simulink model "typMPC"  (R2019b)
settings: Solver=VariableStepAuto  StartTime=0.0  StopTime=10.0  RelTol=1e-3
settings Model: Creator=Daniel  LastModifiedBy=Daniel

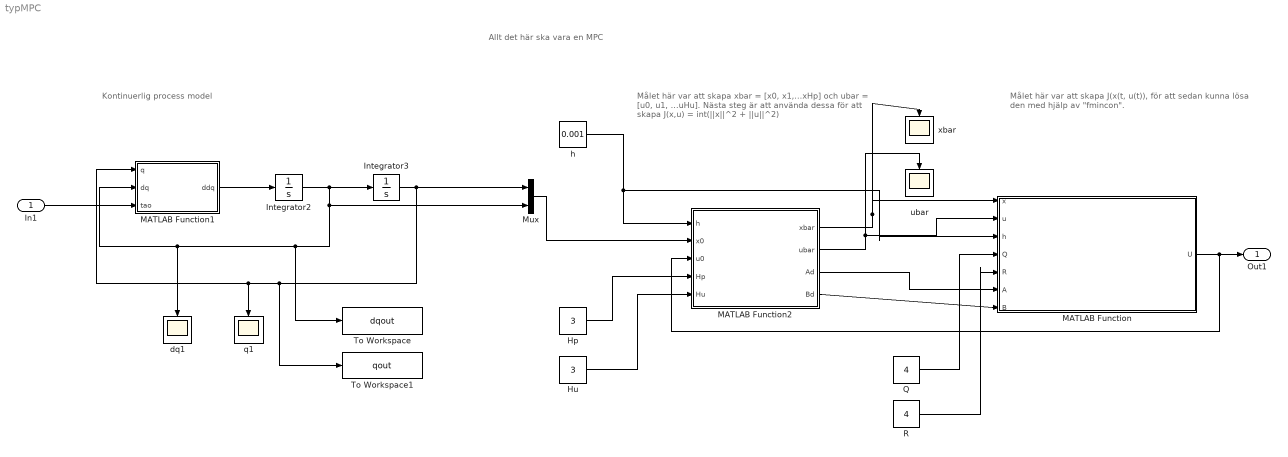
== system typMPC ==
  note: Allt det här ska vara en MPC
  note: Målet här var att skapa J(x(t, u(t)), för att sedan
      | kunna lösa den med hjälp av "fmincon".
  note: Målet här var att skapa xbar = [x0, x1,...xHp]
      | och ubar = [u0, u1, ...uHu].
      | Nästa steg är att använda dessa för att skapa
      | J(x,u) = int(||x||^2 + ||u||^2)
  note: Kontinuerlig process model
  In1 : Inport
  "Hp " : Constant  Value=3
  "Hu " : Constant  Value=3
  Integrator2 : Integrator  InitialCondition=[0;pi/6]
  Integrator3 : Integrator  InitialCondition=[0;0]
  MATLAB Function : MATLAB Function  TreatAsAtomicUnit=on
  MATLAB Function1 : MATLAB Function  TreatAsAtomicUnit=on
  MATLAB Function2 : MATLAB Function  TreatAsAtomicUnit=on
  Mux : Mux  Inputs=2
  Q : Constant  Value=4
  R : Constant  Value=4
  To Workspace : ToWorkspace  VariableName=dqout  SaveFormat=Timeseries  SampleTime=-1
  To Workspace1 : ToWorkspace  VariableName=qout  SampleTime=-1
  dq1 : Scope
  h : Constant  Value=0.001
  q1 : Scope
  ubar : Scope
  xbar : Scope
  Out1 : Outport
  wires:
  MATLAB Function2/2(ubar) -> MATLAB Function/2(u), ubar/1
  Mux/1 -> MATLAB Function2/2(x0)
  "Hu "/1 -> MATLAB Function2/5(Hu)
  MATLAB Function2/1(xbar) -> MATLAB Function/1(x), xbar/1
  "Hp "/1 -> MATLAB Function2/4(Hp)
  h/1 -> MATLAB Function/3(h), MATLAB Function2/1(h)
  Integrator3/1 -> Mux/1, To Workspace1/1, MATLAB Function1/1(q), q1/1
  MATLAB Function1/1(ddq) -> Integrator2/1
  Integrator2/1 -> Mux/2, To Workspace/1, MATLAB Function1/2(dq), dq1/1, Integrator3/1
  MATLAB Function2/3(Ad) -> MATLAB Function/6(A)
  MATLAB Function2/4(Bd) -> MATLAB Function/7(B)
  Q/1 -> MATLAB Function/4(Q)
  R/1 -> MATLAB Function/5(R)
  MATLAB Function/1(U) -> MATLAB Function2/3(u0), Out1/1
  In1/1 -> MATLAB Function1/3(tao)

== matlab function typMPC/MATLAB Function1 ==
  data: q input; ddq output; dq input; tao input
function  ddq  = testing(q,dq,tao)
%% q= [phi, theta],   dq = [dphi, dtheta]
% tao2=[0;tao];
phi = q(1,1);
theta = q(2,1);
dphi = dq(1,1);
dtheta = dq(2,1);
%Given parameters - "competition.pdf"
la  = 75*10^-3;       %[m]      - Length of arm
r  = 43*10^-3;       %[m]      - Base radius
lp  = 31.5*10^-3;     %[m]      - Length of pendulum
J  = 125*10^-6;      %[kgm^2]  - Base moment of inertia
g  = 9.8;            %[m/s^2]  - Gravity
Jc = 2.55*10^-6;     %[kgm^2]  - Moment of inertia of pendulum around c.o.m
M  = 5.44*10^-3;     %[kg]     - Mass of pendulum point mass
Jp = 7.95*10^-6;     %[kgm^2]  - Moment of inertia of pend around pivot

%Still unknown - Try to guess these as a first step
ma = 10*10^-3;       %[kg] - Mass of arm       - Try 10g
mp = 5*10^-3;        %[kg] - Mass of pendulum  - Try 5g

%Equation (17)
global alpha beta gamma delta;
alpha   = J + (M + (1/3)*ma + mp)*la^2;
beta    = (M + (1/3)*mp)*lp^2;
gamma   = (M + (1/2)*mp)*la*lp;
delta   = (M + (1/2)*mp)*g*lp;

D = [(alpha + beta*sin(theta)^2),(gamma*cos(theta));(gamma*cos(theta)),(beta)];
C = [(beta*cos(theta)*sin(theta)*dtheta),(beta*cos(theta)*sin(theta)*dphi - gamma*sin(theta)*dtheta);(-beta*cos(theta)*sin(theta)*dphi),(0)];
G = [0;-delta*sin(theta)];

% ddq = inv(D)*(tao2 - C*dq - G);
ddq = D\(tao2 - C*dq - G);
end

== matlab function typMPC/MATLAB Function2 ==
  data: h input; x0 input; u0 input; xbar output [0..4*Hp]; ubar output; Hp input; Hu input; Ad output; Bd output
function [xbar, ubar, Ad, Bd] = createBars(h, x0, u0, Hp, Hu)
%Input vector xk = [phi_k, dphi_k, theta_k, dtheta_k], and time step h;
%Output vector xk1 = [phi_{k+1}, dphi_{k+1}, theta_{k+1}, dtheta_{k+1}];

%x = [phi, dphi, theta, dtheta]';    %This is the most recent x (x_k)
% x changed to x=[phi,theta,dphi,dtheta]
%Har x0,u0 med i xbar,ubar och u[tao,1] och Bdiskret[B,V].
Hp = Hp+1;
Hu = Hu+1;
if (length(x0) < 4*Hp)
    xbar = zeros(4*Hp,1);
    xbar(1:4) = x0;
else
    xbar = x0;      
end

if (length(u0) < 3*Hu)
    ubar = repmat([0;0;1],Hu,1);
    ubar(1:2) = u0;
else
    ubar = u0;
end
%Vet inte var vi borde införa Xref
Xref=repmat([0;0;0;0],Hp,1);
% phi=xbar(1,1);
theta=xbar(2,1);
dphi=xbar(3,1);
dtheta=xbar(4,1);   
D = [(alpha + beta*sin(theta)^2),(gamma*cos(theta));(gamma*cos(theta)),(beta)];
C = [(beta*cos(theta)*sin(theta)*dtheta),(beta*cos(theta)*sin(theta)*dphi - gamma*sin(theta)*dtheta);(-beta*cos(theta)*sin(theta)*dphi),(0)];
G = [0;-delta*sin(theta)];
f_x = D\(-C -G./x0(3:4));
f_u = D\[1;1];

V1 = x0(1:2)-diag(x0(3:4))*x0(1:2);
A1 = diag(x0(3:4));
B1 = zeros(2,2);
V2 = x0(3:4)-f_x*x0(1:2)-diag(f_u)*u0;
A2 = f_x;
B2= diag(f_u);
Hd =ss([A1,[0,0;0,0];[0,0;0,0],A2],[B1,V1;B2,V2],[0,0,0,0],[],h);
Ad = Hd.A;
Bd = Hd.B;

for i = 2:Hp
    xbar((i*4-3):(i*4)) = xbar((i-1)*4-3:(i-1)*4) + h*(Ad*xbar((i-1)*4-3:(i-1)*4) + Bd*ubar((i-1)*3-2:(i-1)*3));
end

xbar = xbar - Xref;

% % Full model continuous, kommer antagligen vara
% % för resurskrävande att uppdatera matriserna mellan varje iteration.
% dAc = D\(-C -G./x0(3:4));
% dBc = D\[1;1];
% Cc =[0,0];
% Dc =[0];
% Hd = ss(dAc,dBc,Cc,Dc,h);
% dAd = Hd.A;
% dBd = Hd.B;
% 
% for i = 2:Hp
%     xbar((i*4-3):(i*4-2)) = xbar((i-1)*4-3:(i-1)*4-2) + h*(xbar((i-1)*4-1:(i-1)*4));
%     
% %     theta=xbar((i-1)*4-2,1);
% %     dphi=xbar((i-1)*4-1,1);
% %     dtheta=xbar((i-1)*4,1);
% %     D = [(alpha + beta*sin(theta)^2),(gamma*cos(theta));(gamma*cos(theta)),(beta)];
% %     C = [(beta*cos(theta)*sin(theta)*dtheta),(beta*cos(theta)*sin(theta)*dphi - gamma*sin(theta)*dtheta);(-beta*cos(theta)*sin(theta)*dphi),(0)];
% %     G = [0;-delta*sin(theta)];
% %     ddq = D\(-C -G./xbar((i-1)*4-1:(i-1)*4));
% %     xbar((i*4-1):(i*4)) = xbar((i-1)*4-1:(i-1)*4) + h*(ddq*xbar((i-1)*4-1:(i-1)*4) + D\ubar((i-1)*2-1:(i-1)*2));
%     xbar((i*4-1):(i*4)) = xbar((i-1)*4-1:(i-1)*4) + h*(dAd*xbar((i-1)*4-1:(i-1)*4) + dBd*ubar((i-1)*2-1:(i-1)*2));
% end
%%
% Om vi ska ha en linjära diskreta matris A och B, kan vi antingen använda dAd och dBd som
% är baserad på x0 och u0. Det kanske är för resurskrävande att beräkna
% nya ddq varje iteration. Stegen är inte så långa, så det kanske inte
% hinner bli ett så stort fel över Hp. Eller så kan vi fråga marcus om det
% finns en annan approximation vi kan använda.
%% Detta ingår väl i den andra matlab functionen? 
% Ahp = zeros(4*Hp,4*Hp);
% Bhu = zeros(4*Hu,2*Hu);
% for i = 1:Hp
%     Ahp((4*i-3):(4*i), 1:4) = (1+h*A)^i;        %AHp stämmer nog
% end
% Brow = zeros(4, 2*Hu);
% Brow(1:4, 1:2) = h*B;
% Bhu(1:4,:) = Brow;
% for j = 2:Hu
%     Brow = circshift(Brow',2)';
%     Brow(1:4,1:2) = (h*B'*(1+h*A)^(j-1))';
%     Bhu(4*j-3:4*j, :) = Brow;
% end
% 
% xk1 = Ahp(1:4,:)*xbar + Bhu(1:4,:)*ubar;
% xbar(1:4,1) = x0(1:4);
% xbar = circshift(xbar, 4);
% xbar(1:4,1) = xk1(1:4)';
% ubar(1:2, 1) = u0(1:2);
% ubar = circshift(ubar,2);
%Hur ska ubar uppdateras?

end

== matlab function typMPC/MATLAB Function ==
  data: x input; u input; U output; h input; Q input; R input; A input; B input
function U  = solveJacobianVector(x,u,h,Q,R,A,B)
%Try to solve the jacobian J(x,u) = int{||x||^2 + ||u||^2} with fmincon
%The function will return J = [u1(k), u2(k)] which is the optimal
%control law for u, Hu time steps forward in time.
Hp = length(x)/4;           %Prediction Horizon  
Hu = length(u)/2;           %Control Horizon 

%Jag vet inte vÃ¤rdet pÃ¥ A och B. Dessa fÃ¥s frÃ¥n diskretiseringen!
% A = eye(4);                %test - 4*4
% B = ones(4,2);             %test - 4*1

%Constraints for the control signal u - Jag vet inte vad dessa ska va.
% Au = eye(2*Hu);
% Bu = ones(2*Hu,1);
u0 = zeros(2*Hu,1);
                
Mp = zeros(Hp*4, Hu*2);
Np = zeros(4*Hp, 4);
row = zeros(4, Hu*2);
b = (h*B);
a = (1+h*A);
row(1:4,1:2) = b;
for i = 1:Hp
    Mp(4*i-3:4*i,:) = row;
    Np(4*i-3:4*i,:) = a^i;
    row = circshift(row',2)';
    row(1:4,1:2) = (a^i)*b;
end
x = reshape(x, [4,Hp]);

Xk = (Mp*u)+(Np*x(:,1));     %Xk -> (Ekv. 16.40, Rolf Johansson)
Qmat = Q*eye(4*Hp);
Rmat = zeros(2*Hu, 2*Hu);
for k = 1:Hu
    Rmat(k,k) = R;
end
lb=zeros(2*Hu,1);
ub=zeros(2*Hu,1);
for i=1:Hu
    lb(2*i-1:2*i)=[-0.2; -Inf];
    ub(2*i-1:2*i)=[0.2, Inf];
end
Ju = @(uMin)[(Xk'*Qmat*Xk) + [uMin]'*Rmat*[uMin]];
J1 = fmincon(Ju, u0,[],[],[],[],lb,ub);
J = reshape(J1, [2,Hu])';
U=J(:,2);
%% column 1 eller 2(ifall 1 är u0).
end
